simulink model "Bias_TestGen12"  (R2017b)
settings: Solver=FixedStepDiscrete  StartTime=0.0  StopTime=10.0  RelTol=1e-3
undefined symbols (not defined in the file): Block_TestLib, enable_trigger
settings Model: Creator=hbourbou  LastModifiedBy=hbourbou
settings DebuggingCC: ParameterOverflowMsg=none

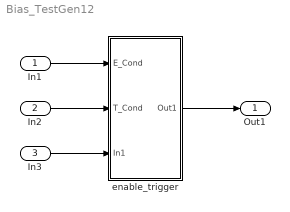
== system Bias_TestGen12 ==
  In1 : Inport
  In2 : Inport  Port=2
  In3 : Inport  Port=3
  enable_trigger : Subsystem  AncestorBlock=Block_TestLib/enable_trigger
  Out1 : Outport
  wires:
  In1/1 -> enable_trigger/1(E_Cond)
  In2/1 -> enable_trigger/2(T_Cond)
  In3/1 -> enable_trigger/3(In1)
  enable_trigger/1(Out1) -> Out1/1

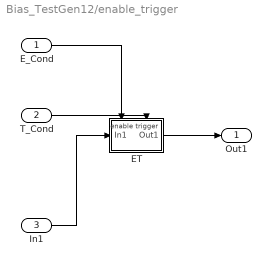
== system Bias_TestGen12/enable_trigger ==
  E_Cond : Inport  OutDataTypeStr=boolean
  T_Cond : Inport  Port=2  OutDataTypeStr=boolean
  In1 : Inport  Port=3
  ET : Subsystem  TreatAsAtomicUnit=on
  Out1 : Outport
  wires:
  T_Cond/1 -> ET/Trigger
  E_Cond/1 -> ET/Enable
  In1/1 -> ET/1(In1)
  ET/1(Out1) -> Out1/1

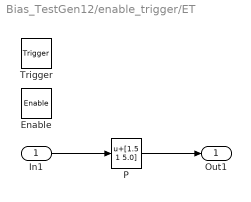
== system Bias_TestGen12/enable_trigger/ET ==
  In1 : Inport  OutDataTypeStr=int16  PortDimensions=[1 3]
  Enable : EnablePort
  Trigger : TriggerPort  VariantControl=Variant
  P : Bias  Bias=[1.5 1 5.0]  SaturateOnIntegerOverflow=on
  Out1 : Outport
  wires:
  In1/1 -> P/1
  P/1 -> Out1/1
